simulink model "simulretardordre2"  (R2022a)
settings: Solver=VariableStepAuto  StartTime=0.0  StopTime=100  RelTol=1e-3
libraries: simulink x2
settings Model: Creator=alexa  LastModifiedBy=alexa
settings DebuggingCC: UnconnectedInputMsg=warning  UnconnectedOutputMsg=warning  UnconnectedLineMsg=warning
settings RTWCC: DLArmComputeVersion=19.05

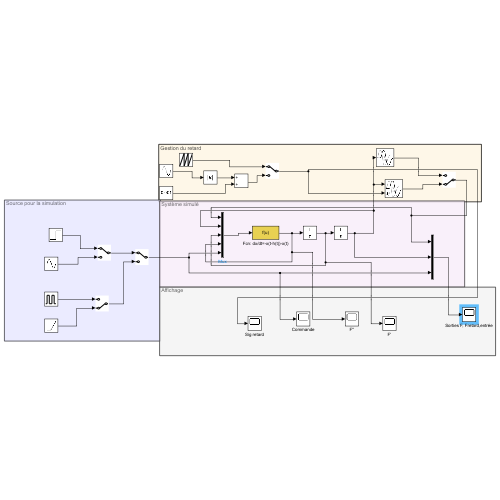
[thumbnail: Simulink's stored preview of the top-level diagram]
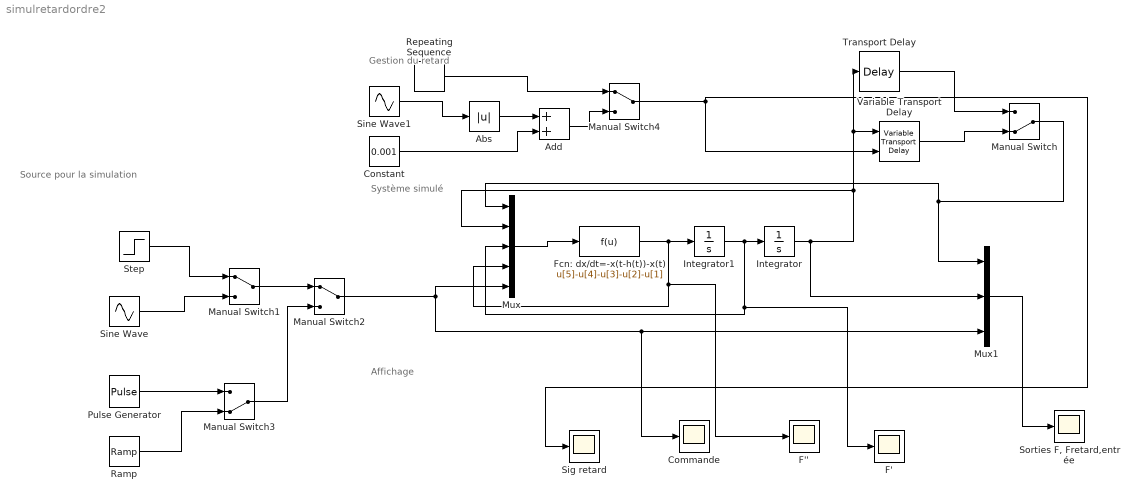
== system simulretardordre2 ==
  note: Affichage
  note: Système simulé
  note: Gestion du retard
  note: Source pour la simulation
  Abs : Abs  SaturateOnIntegerOverflow=off
  Add : Sum
  Commande : Scope
  Constant : Constant  Value=0.001
  F' : Scope
  F'' : Scope
  Fcn: dx/dt=-x(t-h(t))-x(t) : Fcn  Expr=u[5]-u[4]-u[3]-u[2]-u[1]
  Integrator : Integrator
  Integrator1 : Integrator
  Manual Switch : ManualSwitch  CurrentSetting=0
  Manual Switch1 : ManualSwitch
  Manual Switch2 : ManualSwitch
  Manual Switch3 : ManualSwitch  CurrentSetting=0
  Manual Switch4 : ManualSwitch
  Mux : Mux  Inputs=5
  Mux1 : Mux  Inputs=3
  Pulse Generator : DiscretePulseGenerator  PulseType=Time based  Amplitude=10  Period=10  PulseWidth=75  PhaseDelay=1
  Ramp : simulink/Sources/Ramp  slope=1  start=0  InitialOutput=0
  Repeating Sequence : simulink/Sources/Repeating Sequence  rep_seq_t=[0 5]  rep_seq_y=[0.1 3]
  Sig retard : Scope
  Sine Wave : Sin  Amplitude=10  SampleTime=0
  Sine Wave1 : Sin  SineType=Sample based  Amplitude=2  Frequency=0.3*2*pi  Samples=100  SampleTime=0.01  Offset=1
  "Sorties F, Fretard,entrée" : Scope
      settings: Tag=Scope retard
  Step : Step  After=10  SampleTime=0
  Transport Delay : TransportDelay  DelayTime=5
  Variable Transport Delay : VariableTransportDelay  VariableDelayType=Variable transport delay  MaximumDelay=15
  wires:
  Mux/1 -> Fcn: dx/dt=-x(t-h(t))-x(t)/1
  Fcn: dx/dt=-x(t-h(t))-x(t)/1 -> Integrator1/1, Mux/4, F''/1
  Integrator/1 -> Mux1/2, Mux/2, Transport Delay/1, Variable Transport Delay/1
  Mux1/1 -> "Sorties F, Fretard,entrée"/1
  Transport Delay/1 -> Manual Switch/1
  Variable Transport Delay/1 -> Manual Switch/2
  Manual Switch/1 -> Mux1/1, Mux/1
  Step/1 -> Manual Switch1/1
  Sine Wave/1 -> Manual Switch1/2
  Manual Switch1/1 -> Manual Switch2/1
  Manual Switch2/1 -> Commande/1, Mux1/3, Mux/5
  Pulse Generator/1 -> Manual Switch3/1
  Ramp/1 -> Manual Switch3/2
  Manual Switch3/1 -> Manual Switch2/2
  Repeating Sequence/1 -> Manual Switch4/1
  Manual Switch4/1 -> Sig retard/1, Variable Transport Delay/2
  Sine Wave1/1 -> Abs/1
  Constant/1 -> Add/2
  Abs/1 -> Add/1
  Add/1 -> Manual Switch4/2
  Integrator1/1 -> F'/1, Mux/3, Integrator/1
